simulink library "inp"  (R2021b)
settings: Solver=VariableStepAuto  StartTime=0.0  StopTime=10.0  RelTol=1e-3
undefined symbols (not defined in the file): C_TASK_5MS_S, FALSE, KINP_AcoreReadyToSlp_flg_ovrdflg, KINP_AcoreReadyToSlp_flg_ovrdval, KINP_AllowMovThd_OTA_enum_ovrdflg, KINP_AllowMovThd_OTA_enum_ovrdval, KINP_APSAngleTarget_Deg_ovrdflg, KINP_APSAngleTarget_Deg_ovrdval, KINP_APSDecReq_mps2_ovrdflg, KINP_APSDecReq_mps2_ovrdval, KINP_APSDecReqA_flg_ovrdflg, KINP_APSDecReqA_flg_ovrdval, KINP_APSDFLL_cm_ovrdflg, KINP_APSDFLL_cm_ovrdval, KINP_APSDFLR_cm_ovrdflg, KINP_APSDFLR_cm_ovrdval, KINP_APSDRLL_cm_ovrdflg, KINP_APSDRLL_cm_ovrdval, KINP_APSDRLR_cm_ovrdflg, KINP_APSDRLR_cm_ovrdval, KINP_APSExitCondition_enum_ovrdflg, KINP_APSExitCondition_enum_ovrdval, KINP_APSHWVer_enum_ovrdflg, KINP_APSHWVer_enum_ovrdval, KINP_APSProgressPCT_pct_ovrdflg, KINP_APSProgressPCT_pct_ovrdval, KINP_APSReq_enum_ovrdflg, KINP_APSReq_enum_ovrdval, KINP_APSRQDisplay_enum_ovrdflg, KINP_APSRQDisplay_enum_ovrdval, KINP_APSRqEPASCtrl_flg_ovrdflg, KINP_APSRqEPASCtrl_flg_ovrdval, KINP_APSShiftPosnReq_enum_ovrdval, KINP_APSShiftPosnReq_enum_ovrflg, KINP_APSSpeedCMD_kph_ovrdval, KINP_APSSpeedCMD_kph_ovrflg, KINP_APSStaSystem_enum_ovrdflg, KINP_APSStaSystem_enum_ovrdval, KINP_APSSWVer_enum_ovrdflg, KINP_APSSWVer_enum_ovrdval, KINP_APSVMCReqA_flg_ovrdval, KINP_APSVMCReqA_flg_ovrflg, KINP_APSVRqEPASCtrl_flg_ovrdflg, KINP_APSVRqEPASCtrl_flg_ovrdval, KINP_AuxBattVolmV_mV_ovrdflg, KINP_AuxBattVolmV_mV_ovrdval, KINP_CAASSta_enum_ovrdflg, KINP_CAASSta_enum_ovrdval, KINP_CAASVMCReqA_flg_ovrdval, KINP_CAASVMCReqA_flg_ovrflg, KINP_Chime_enum_ovrdflg, KINP_Chime_enum_ovrdval, KINP_ClearDTCcmd_flg_ovrdflg, KINP_ClearDTCcmd_flg_ovrdval, KINP_EvccAplusPwrUpReq_flg_ovrdflg, KINP_EvccAplusPwrUpReq_flg_ovrdval, KINP_LFID_raw_ovrdval, KINP_LFID_raw_ovrflg, KINP_LRID_raw_ovrdval, KINP_MemOffsetAccX_raw16_ovrdflg ... (+118)
libraries: FVT_lib x595, hcu_lib x1
(part 24 of 27)

== system inp/INP/CAN4/SignalCheck/GW_ZoneFR2 ==
  BHAL_outputs : Inport
  inp_CanValid_bus : Inport  Port=2
  COMPStatorSpd : FVT_lib/inp/can_signal_template  SystemSampleTime=-1  VariantActivationTime=update diagram  Latency=0  AutoFrameSizeCalculation=off
      link override defval: Value=KINP_COMPStatorSpd_rpm_defval
      link override fftdec: Value=KINP_COMPStatorSpd_rpm_fftdec
      link override fftinc: Value=KINP_COMPStatorSpd_rpm_fftinc
      link override fftlim: Value=KINP_COMPStatorSpd_rpm_fftlim
      link override invalid: Value=KINP_COMPStatorSpd_rpm_invalid
      link override ovrdflg: Value=KINP_COMPStatorSpd_rpm_ovrdflg
      link override ovrdval: Value=KINP_COMPStatorSpd_rpm_ovrdval
      link override setvalid: Value=KINP_COMPStatorSpd_rpm_setvalid
      link override srvcflg: Value=KINP_COMPStatorSpd_rpm_srvcflg
      link override srvcval: Value=KINP_COMPStatorSpd_rpm_srvcval
  CompProEN : FVT_lib/inp/can_signal_template  SystemSampleTime=-1  VariantActivationTime=update diagram  Latency=0  AutoFrameSizeCalculation=off
      link override defval: Value=KINP_CompProEN_flg_defval
      link override fftdec: Value=KINP_CompProEN_flg_fftdec
      link override fftinc: Value=KINP_CompProEN_flg_fftinc
      link override fftlim: Value=KINP_CompProEN_flg_fftlim
      link override invalid: Value=KINP_CompProEN_flg_invalid
      link override ovrdflg: Value=KINP_CompProEN_flg_ovrdflg
      link override ovrdval: Value=KINP_CompProEN_flg_ovrdval
      link override setvalid: Value=KINP_CompProEN_flg_setvalid
      link override srvcflg: Value=KINP_CompProEN_flg_srvcflg
      link override srvcval: Value=KINP_CompProEN_flg_srvcval
  Terminator_1 : Terminator
  Terminator_2 : Terminator
  True_VHAL_COMPStatorSpd_rpm : Constant  Value=TRUE  OutDataTypeStr=boolean
  True_VHAL_CompProEN_flg : Constant  Value=TRUE  OutDataTypeStr=boolean
  slr1_1 : BusSelector  OutputSignals=VINP_CANMsgValidGWZoneFR2_flg
  slr1_2 : BusSelector  OutputSignals=VINP_CANMsgValidGWZoneFR2_flg
  slr_VHAL_COMPStatorSpd_rpm : BusSelector  OutputSignals=VHAL_COMPStatorSpd_rpm
  slr_VHAL_CompProEN_flg : BusSelector  OutputSignals=VHAL_CompProEN_flg
  VINP_COMPStatorSpd_rpm : Outport
  VINP_CompProEN_flg : Outport  Port=2
  wires:
  BHAL_outputs/1 -> [BHAL_outputs]
  inp_CanValid_bus/1 -> [inp_CanValid_bus]
  [BHAL_outputs] -> slr_VHAL_COMPStatorSpd_rpm/1
  slr_VHAL_COMPStatorSpd_rpm/1 -> COMPStatorSpd/1  "<VHAL_COMPStatorSpd_rpm>"
  True_VHAL_COMPStatorSpd_rpm/1 -> COMPStatorSpd/2
  [inp_CanValid_bus] -> slr1_1/1
  slr1_1/1 -> COMPStatorSpd/3  "<VINP_CANMsgValidGWZoneFR2_flg>"
  COMPStatorSpd/1 -> VINP_COMPStatorSpd_rpm/1  "VINP_COMPStatorSpd_rpm"
  COMPStatorSpd/2 -> Terminator_1/1
  [BHAL_outputs] -> slr_VHAL_CompProEN_flg/1
  slr_VHAL_CompProEN_flg/1 -> CompProEN/1  "<VHAL_CompProEN_flg>"
  True_VHAL_CompProEN_flg/1 -> CompProEN/2
  [inp_CanValid_bus] -> slr1_2/1
  slr1_2/1 -> CompProEN/3  "<VINP_CANMsgValidGWZoneFR2_flg>"
  CompProEN/1 -> VINP_CompProEN_flg/1  "VINP_CompProEN_flg"
  CompProEN/2 -> Terminator_2/1

== system inp/INP/CAN4/SignalCheck/Zone_Dr_SCP ==
  BHAL_outputs : Inport
  inp_CanValid_bus : Inport  Port=2
  DrSCPSysErrLmp : FVT_lib/inp/can_signal_template  SystemSampleTime=-1  VariantActivationTime=update diagram  Latency=0  AutoFrameSizeCalculation=off
      link override defval: Value=KINP_DrSCPSysErrLmp_flg_defval
      link override fftdec: Value=KINP_DrSCPSysErrLmp_flg_fftdec
      link override fftinc: Value=KINP_DrSCPSysErrLmp_flg_fftinc
      link override fftlim: Value=KINP_DrSCPSysErrLmp_flg_fftlim
      link override invalid: Value=KINP_DrSCPSysErrLmp_flg_invalid
      link override ovrdflg: Value=KINP_DrSCPSysErrLmp_flg_ovrdflg
      link override ovrdval: Value=KINP_DrSCPSysErrLmp_flg_ovrdval
      link override setvalid: Value=KINP_DrSCPSysErrLmp_flg_setvalid
      link override srvcflg: Value=KINP_DrSCPSysErrLmp_flg_srvcflg
      link override srvcval: Value=KINP_DrSCPSysErrLmp_flg_srvcval
  RegenMode : FVT_lib/inp/can_signal_template  SystemSampleTime=-1  VariantActivationTime=update diagram  Latency=0  AutoFrameSizeCalculation=off
      link override defval: Value=KINP_RegenMode_enum_defval
      link override fftdec: Value=KINP_RegenMode_enum_fftdec
      link override fftinc: Value=KINP_RegenMode_enum_fftinc
      link override fftlim: Value=KINP_RegenMode_enum_fftlim
      link override invalid: Value=KINP_RegenMode_enum_invalid
      link override ovrdflg: Value=KINP_RegenMode_enum_ovrdflg
      link override ovrdval: Value=KINP_RegenMode_enum_ovrdval
      link override setvalid: Value=KINP_RegenMode_enum_setvalid
      link override srvcflg: Value=KINP_RegenMode_enum_srvcflg
      link override srvcval: Value=KINP_RegenMode_enum_srvcval
  SetSpd : FVT_lib/inp/can_signal_template  SystemSampleTime=-1  VariantActivationTime=update diagram  Latency=0  AutoFrameSizeCalculation=off
      link override defval: Value=KINP_SetSpd_kph_defval
      link override fftdec: Value=KINP_SetSpd_kph_fftdec
      link override fftinc: Value=KINP_SetSpd_kph_fftinc
      link override fftlim: Value=KINP_SetSpd_kph_fftlim
      link override invalid: Value=KINP_SetSpd_kph_invalid
      link override ovrdflg: Value=KINP_SetSpd_kph_ovrdflg
      link override ovrdval: Value=KINP_SetSpd_kph_ovrdval
      link override setvalid: Value=KINP_SetSpd_kph_setvalid
      link override srvcflg: Value=KINP_SetSpd_kph_srvcflg
      link override srvcval: Value=KINP_SetSpd_kph_srvcval
  Terminator_{1..4} (4 alike) : Terminator
  True_VHAL_DrSCPSysErrLmp_flg : Constant  Value=TRUE  OutDataTypeStr=boolean
  True_VHAL_RegenMode_enum : Constant  Value=TRUE  OutDataTypeStr=boolean
  True_VHAL_SetSpd_kph : Constant  Value=TRUE  OutDataTypeStr=boolean
  True_VHAL_ZoneSpdCtrlMode_enum : Constant  Value=TRUE  OutDataTypeStr=boolean
  ZoneSpdCtrlMode : FVT_lib/inp/can_signal_template  SystemSampleTime=-1  VariantActivationTime=update diagram  Latency=0  AutoFrameSizeCalculation=off
      link override defval: Value=KINP_ZoneSpdCtrlMode_enum_defval
      link override fftdec: Value=KINP_ZoneSpdCtrlMode_enum_fftdec
      link override fftinc: Value=KINP_ZoneSpdCtrlMode_enum_fftinc
      link override fftlim: Value=KINP_ZoneSpdCtrlMode_enum_fftlim
      link override invalid: Value=KINP_ZoneSpdCtrlMode_enum_invalid
      link override ovrdflg: Value=KINP_ZoneSpdCtrlMode_enum_ovrdflg
      link override ovrdval: Value=KINP_ZoneSpdCtrlMode_enum_ovrdval
      link override setvalid: Value=KINP_ZoneSpdCtrlMode_enum_setvalid
      link override srvcflg: Value=KINP_ZoneSpdCtrlMode_enum_srvcflg
      link override srvcval: Value=KINP_ZoneSpdCtrlMode_enum_srvcval
  slr1_{1..4} (4 alike) : BusSelector  OutputSignals=VINP_CANMsgValidZoneDrSCP_flg
  slr_VHAL_DrSCPSysErrLmp_flg : BusSelector  OutputSignals=VHAL_DrSCPSysErrLmp_flg
  slr_VHAL_RegenMode_enum : BusSelector  OutputSignals=VHAL_RegenMode_enum
  slr_VHAL_SetSpd_kph : BusSelector  OutputSignals=VHAL_SetSpd_kph
  slr_VHAL_ZoneSpdCtrlMode_enum : BusSelector  OutputSignals=VHAL_ZoneSpdCtrlMode_enum
  VINP_DrSCPSysErrLmp_flg : Outport
  VINP_RegenMode_enum : Outport  Port=2
  VINP_SetSpd_kph : Outport  Port=3
  VINP_ZoneSpdCtrlMode_enum : Outport  Port=4
  wires:
  BHAL_outputs/1 -> [BHAL_outputs]
  inp_CanValid_bus/1 -> [inp_CanValid_bus]
  [BHAL_outputs] -> slr_VHAL_DrSCPSysErrLmp_flg/1
  slr_VHAL_DrSCPSysErrLmp_flg/1 -> DrSCPSysErrLmp/1  "<VHAL_DrSCPSysErrLmp_flg>"
  True_VHAL_DrSCPSysErrLmp_flg/1 -> DrSCPSysErrLmp/2
  [inp_CanValid_bus] -> slr1_1/1
  slr1_1/1 -> DrSCPSysErrLmp/3  "<VINP_CANMsgValidZoneDrSCP_flg>"
  DrSCPSysErrLmp/1 -> VINP_DrSCPSysErrLmp_flg/1  "VINP_DrSCPSysErrLmp_flg"
  DrSCPSysErrLmp/2 -> Terminator_1/1
  [BHAL_outputs] -> slr_VHAL_RegenMode_enum/1
  slr_VHAL_RegenMode_enum/1 -> RegenMode/1  "<VHAL_RegenMode_enum>"
  True_VHAL_RegenMode_enum/1 -> RegenMode/2
  [inp_CanValid_bus] -> slr1_2/1
  slr1_2/1 -> RegenMode/3  "<VINP_CANMsgValidZoneDrSCP_flg>"
  RegenMode/1 -> VINP_RegenMode_enum/1  "VINP_RegenMode_enum"
  RegenMode/2 -> Terminator_2/1
  [BHAL_outputs] -> slr_VHAL_SetSpd_kph/1
  slr_VHAL_SetSpd_kph/1 -> SetSpd/1  "<VHAL_SetSpd_kph>"
  True_VHAL_SetSpd_kph/1 -> SetSpd/2
  [inp_CanValid_bus] -> slr1_3/1
  slr1_3/1 -> SetSpd/3  "<VINP_CANMsgValidZoneDrSCP_flg>"
  SetSpd/1 -> VINP_SetSpd_kph/1  "VINP_SetSpd_kph"
  SetSpd/2 -> Terminator_3/1
  [BHAL_outputs] -> slr_VHAL_ZoneSpdCtrlMode_enum/1
  slr_VHAL_ZoneSpdCtrlMode_enum/1 -> ZoneSpdCtrlMode/1  "<VHAL_ZoneSpdCtrlMode_enum>"
  True_VHAL_ZoneSpdCtrlMode_enum/1 -> ZoneSpdCtrlMode/2
  [inp_CanValid_bus] -> slr1_4/1
  slr1_4/1 -> ZoneSpdCtrlMode/3  "<VINP_CANMsgValidZoneDrSCP_flg>"
  ZoneSpdCtrlMode/1 -> VINP_ZoneSpdCtrlMode_enum/1  "VINP_ZoneSpdCtrlMode_enum"
  ZoneSpdCtrlMode/2 -> Terminator_4/1

== system inp/INP/CAN4/SignalCheck/Zone_Dr_THCM ==
  BHAL_outputs : Inport
  inp_CanValid_bus : Inport  Port=2
  BlowerErr : FVT_lib/inp/can_signal_template  SystemSampleTime=-1  VariantActivationTime=update diagram  Latency=0  AutoFrameSizeCalculation=off
      link override defval: Value=KINP_BlowerErr_enum_defval
      link override fftdec: Value=KINP_BlowerErr_enum_fftdec
      link override fftinc: Value=KINP_BlowerErr_enum_fftinc
      link override fftlim: Value=KINP_BlowerErr_enum_fftlim
      link override invalid: Value=KINP_BlowerErr_enum_invalid
      link override ovrdflg: Value=KINP_BlowerErr_enum_ovrdflg
      link override ovrdval: Value=KINP_BlowerErr_enum_ovrdval
      link override setvalid: Value=KINP_BlowerErr_enum_setvalid
      link override srvcflg: Value=KINP_BlowerErr_enum_srvcflg
      link override srvcval: Value=KINP_BlowerErr_enum_srvcval
  SolarL : FVT_lib/inp/can_signal_template  SystemSampleTime=-1  VariantActivationTime=update diagram  Latency=0  AutoFrameSizeCalculation=off
      link override defval: Value=KINP_SolarL_W_defval
      link override fftdec: Value=KINP_SolarL_W_fftdec
      link override fftinc: Value=KINP_SolarL_W_fftinc
      link override fftlim: Value=KINP_SolarL_W_fftlim
      link override invalid: Value=KINP_SolarL_W_invalid
      link override ovrdflg: Value=KINP_SolarL_W_ovrdflg
      link override ovrdval: Value=KINP_SolarL_W_ovrdval
      link override setvalid: Value=KINP_SolarL_W_setvalid
      link override srvcflg: Value=KINP_SolarL_W_srvcflg
      link override srvcval: Value=KINP_SolarL_W_srvcval
  SolarLErr : FVT_lib/inp/can_signal_template  SystemSampleTime=-1  VariantActivationTime=update diagram  Latency=0  AutoFrameSizeCalculation=off
      link override defval: Value=KINP_SolarLErr_enum_defval
      link override fftdec: Value=KINP_SolarLErr_enum_fftdec
      link override fftinc: Value=KINP_SolarLErr_enum_fftinc
      link override fftlim: Value=KINP_SolarLErr_enum_fftlim
      link override invalid: Value=KINP_SolarLErr_enum_invalid
      link override ovrdflg: Value=KINP_SolarLErr_enum_ovrdflg
      link override ovrdval: Value=KINP_SolarLErr_enum_ovrdval
      link override setvalid: Value=KINP_SolarLErr_enum_setvalid
      link override srvcflg: Value=KINP_SolarLErr_enum_srvcflg
      link override srvcval: Value=KINP_SolarLErr_enum_srvcval
  SolarR : FVT_lib/inp/can_signal_template  SystemSampleTime=-1  VariantActivationTime=update diagram  Latency=0  AutoFrameSizeCalculation=off
      link override defval: Value=KINP_SolarR_W_defval
      link override fftdec: Value=KINP_SolarR_W_fftdec
      link override fftinc: Value=KINP_SolarR_W_fftinc
      link override fftlim: Value=KINP_SolarR_W_fftlim
      link override invalid: Value=KINP_SolarR_W_invalid
      link override ovrdflg: Value=KINP_SolarR_W_ovrdflg
      link override ovrdval: Value=KINP_SolarR_W_ovrdval
      link override setvalid: Value=KINP_SolarR_W_setvalid
      link override srvcflg: Value=KINP_SolarR_W_srvcflg
      link override srvcval: Value=KINP_SolarR_W_srvcval
  SolarRErr : FVT_lib/inp/can_signal_template  SystemSampleTime=-1  VariantActivationTime=update diagram  Latency=0  AutoFrameSizeCalculation=off
      link override defval: Value=KINP_SolarRErr_enum_defval
      link override fftdec: Value=KINP_SolarRErr_enum_fftdec
      link override fftinc: Value=KINP_SolarRErr_enum_fftinc
      link override fftlim: Value=KINP_SolarRErr_enum_fftlim
      link override invalid: Value=KINP_SolarRErr_enum_invalid
      link override ovrdflg: Value=KINP_SolarRErr_enum_ovrdflg
      link override ovrdval: Value=KINP_SolarRErr_enum_ovrdval
      link override setvalid: Value=KINP_SolarRErr_enum_setvalid
      link override srvcflg: Value=KINP_SolarRErr_enum_srvcflg
      link override srvcval: Value=KINP_SolarRErr_enum_srvcval
  TFaceL : FVT_lib/inp/can_signal_template  SystemSampleTime=-1  VariantActivationTime=update diagram  Latency=0  AutoFrameSizeCalculation=off
      link override defval: Value=KINP_TFaceL_C_defval
      link override fftdec: Value=KINP_TFaceL_C_fftdec
      link override fftinc: Value=KINP_TFaceL_C_fftinc
      link override fftlim: Value=KINP_TFaceL_C_fftlim
      link override invalid: Value=KINP_TFaceL_C_invalid
      link override ovrdflg: Value=KINP_TFaceL_C_ovrdflg
      link override ovrdval: Value=KINP_TFaceL_C_ovrdval
      link override setvalid: Value=KINP_TFaceL_C_setvalid
      link override srvcflg: Value=KINP_TFaceL_C_srvcflg
      link override srvcval: Value=KINP_TFaceL_C_srvcval
  TFaceLErr : FVT_lib/inp/can_signal_template  SystemSampleTime=-1  VariantActivationTime=update diagram  Latency=0  AutoFrameSizeCalculation=off
      link override defval: Value=KINP_TFaceLErr_enum_defval
      link override fftdec: Value=KINP_TFaceLErr_enum_fftdec
      link override fftinc: Value=KINP_TFaceLErr_enum_fftinc
      link override fftlim: Value=KINP_TFaceLErr_enum_fftlim
      link override invalid: Value=KINP_TFaceLErr_enum_invalid
      link override ovrdflg: Value=KINP_TFaceLErr_enum_ovrdflg
      link override ovrdval: Value=KINP_TFaceLErr_enum_ovrdval
      link override setvalid: Value=KINP_TFaceLErr_enum_setvalid
      link override srvcflg: Value=KINP_TFaceLErr_enum_srvcflg
      link override srvcval: Value=KINP_TFaceLErr_enum_srvcval
  TFaceR : FVT_lib/inp/can_signal_template  SystemSampleTime=-1  VariantActivationTime=update diagram  Latency=0  AutoFrameSizeCalculation=off
      link override defval: Value=KINP_TFaceR_C_defval
      link override fftdec: Value=KINP_TFaceR_C_fftdec
      link override fftinc: Value=KINP_TFaceR_C_fftinc
      link override fftlim: Value=KINP_TFaceR_C_fftlim
      link override invalid: Value=KINP_TFaceR_C_invalid
      link override ovrdflg: Value=KINP_TFaceR_C_ovrdflg
      link override ovrdval: Value=KINP_TFaceR_C_ovrdval
      link override setvalid: Value=KINP_TFaceR_C_setvalid
      link override srvcflg: Value=KINP_TFaceR_C_srvcflg
      link override srvcval: Value=KINP_TFaceR_C_srvcval
  TFaceRErr : FVT_lib/inp/can_signal_template  SystemSampleTime=-1  VariantActivationTime=update diagram  Latency=0  AutoFrameSizeCalculation=off
      link override defval: Value=KINP_TFaceRErr_enum_defval
      link override fftdec: Value=KINP_TFaceRErr_enum_fftdec
      link override fftinc: Value=KINP_TFaceRErr_enum_fftinc
      link override fftlim: Value=KINP_TFaceRErr_enum_fftlim
      link override invalid: Value=KINP_TFaceRErr_enum_invalid
      link override ovrdflg: Value=KINP_TFaceRErr_enum_ovrdflg
      link override ovrdval: Value=KINP_TFaceRErr_enum_ovrdval
      link override setvalid: Value=KINP_TFaceRErr_enum_setvalid
      link override srvcflg: Value=KINP_TFaceRErr_enum_srvcflg
      link override srvcval: Value=KINP_TFaceRErr_enum_srvcval
  TFaceRr : FVT_lib/inp/can_signal_template  SystemSampleTime=-1  VariantActivationTime=update diagram  Latency=0  AutoFrameSizeCalculation=off
      link override defval: Value=KINP_TFaceRr_C_defval
      link override fftdec: Value=KINP_TFaceRr_C_fftdec
      link override fftinc: Value=KINP_TFaceRr_C_fftinc
      link override fftlim: Value=KINP_TFaceRr_C_fftlim
      link override invalid: Value=KINP_TFaceRr_C_invalid
      link override ovrdflg: Value=KINP_TFaceRr_C_ovrdflg
      link override ovrdval: Value=KINP_TFaceRr_C_ovrdval
      link override setvalid: Value=KINP_TFaceRr_C_setvalid
      link override srvcflg: Value=KINP_TFaceRr_C_srvcflg
      link override srvcval: Value=KINP_TFaceRr_C_srvcval
  TFaceRrErr : FVT_lib/inp/can_signal_template  SystemSampleTime=-1  VariantActivationTime=update diagram  Latency=0  AutoFrameSizeCalculation=off
      link override defval: Value=KINP_TFaceRrErr_enum_defval
      link override fftdec: Value=KINP_TFaceRrErr_enum_fftdec
      link override fftinc: Value=KINP_TFaceRrErr_enum_fftinc
      link override fftlim: Value=KINP_TFaceRrErr_enum_fftlim
      link override invalid: Value=KINP_TFaceRrErr_enum_invalid
      link override ovrdflg: Value=KINP_TFaceRrErr_enum_ovrdflg
      link override ovrdval: Value=KINP_TFaceRrErr_enum_ovrdval
      link override setvalid: Value=KINP_TFaceRrErr_enum_setvalid
      link override srvcflg: Value=KINP_TFaceRrErr_enum_srvcflg
      link override srvcval: Value=KINP_TFaceRrErr_enum_srvcval
  TFootL : FVT_lib/inp/can_signal_template  SystemSampleTime=-1  VariantActivationTime=update diagram  Latency=0  AutoFrameSizeCalculation=off
      link override defval: Value=KINP_TFootL_C_defval
      link override fftdec: Value=KINP_TFootL_C_fftdec
      link override fftinc: Value=KINP_TFootL_C_fftinc
      link override fftlim: Value=KINP_TFootL_C_fftlim
      link override invalid: Value=KINP_TFootL_C_invalid
      link override ovrdflg: Value=KINP_TFootL_C_ovrdflg
      link override ovrdval: Value=KINP_TFootL_C_ovrdval
      link override setvalid: Value=KINP_TFootL_C_setvalid
      link override srvcflg: Value=KINP_TFootL_C_srvcflg
      link override srvcval: Value=KINP_TFootL_C_srvcval
  TFootLErr : FVT_lib/inp/can_signal_template  SystemSampleTime=-1  VariantActivationTime=update diagram  Latency=0  AutoFrameSizeCalculation=off
      link override defval: Value=KINP_TFootLErr_enum_defval
      link override fftdec: Value=KINP_TFootLErr_enum_fftdec
      link override fftinc: Value=KINP_TFootLErr_enum_fftinc
      link override fftlim: Value=KINP_TFootLErr_enum_fftlim
      link override invalid: Value=KINP_TFootLErr_enum_invalid
      link override ovrdflg: Value=KINP_TFootLErr_enum_ovrdflg
      link override ovrdval: Value=KINP_TFootLErr_enum_ovrdval
      link override setvalid: Value=KINP_TFootLErr_enum_setvalid
      link override srvcflg: Value=KINP_TFootLErr_enum_srvcflg
      link override srvcval: Value=KINP_TFootLErr_enum_srvcval
  TFootR : FVT_lib/inp/can_signal_template  SystemSampleTime=-1  VariantActivationTime=update diagram  Latency=0  AutoFrameSizeCalculation=off
      link override defval: Value=KINP_TFootR_C_defval
      link override fftdec: Value=KINP_TFootR_C_fftdec
      link override fftinc: Value=KINP_TFootR_C_fftinc
      link override fftlim: Value=KINP_TFootR_C_fftlim
      link override invalid: Value=KINP_TFootR_C_invalid
      link override ovrdflg: Value=KINP_TFootR_C_ovrdflg
      link override ovrdval: Value=KINP_TFootR_C_ovrdval
      link override setvalid: Value=KINP_TFootR_C_setvalid
      link override srvcflg: Value=KINP_TFootR_C_srvcflg
      link override srvcval: Value=KINP_TFootR_C_srvcval
  TFootRErr : FVT_lib/inp/can_signal_template  SystemSampleTime=-1  VariantActivationTime=update diagram  Latency=0  AutoFrameSizeCalculation=off
      link override defval: Value=KINP_TFootRErr_enum_defval
      link override fftdec: Value=KINP_TFootRErr_enum_fftdec
      link override fftinc: Value=KINP_TFootRErr_enum_fftinc
      link override fftlim: Value=KINP_TFootRErr_enum_fftlim
      link override invalid: Value=KINP_TFootRErr_enum_invalid
      link override ovrdflg: Value=KINP_TFootRErr_enum_ovrdflg
      link override ovrdval: Value=KINP_TFootRErr_enum_ovrdval
      link override setvalid: Value=KINP_TFootRErr_enum_setvalid
      link override srvcflg: Value=KINP_TFootRErr_enum_srvcflg
      link override srvcval: Value=KINP_TFootRErr_enum_srvcval
  TFootRr : FVT_lib/inp/can_signal_template  SystemSampleTime=-1  VariantActivationTime=update diagram  Latency=0  AutoFrameSizeCalculation=off
      link override defval: Value=KINP_TFootRr_C_defval
      link override fftdec: Value=KINP_TFootRr_C_fftdec
      link override fftinc: Value=KINP_TFootRr_C_fftinc
      link override fftlim: Value=KINP_TFootRr_C_fftlim
      link override invalid: Value=KINP_TFootRr_C_invalid
      link override ovrdflg: Value=KINP_TFootRr_C_ovrdflg
      link override ovrdval: Value=KINP_TFootRr_C_ovrdval
      link override setvalid: Value=KINP_TFootRr_C_setvalid
      link override srvcflg: Value=KINP_TFootRr_C_srvcflg
      link override srvcval: Value=KINP_TFootRr_C_srvcval
  TFootRrErr : FVT_lib/inp/can_signal_template  SystemSampleTime=-1  VariantActivationTime=update diagram  Latency=0  AutoFrameSizeCalculation=off
      link override defval: Value=KINP_TFootRrErr_enum_defval
      link override fftdec: Value=KINP_TFootRrErr_enum_fftdec
      link override fftinc: Value=KINP_TFootRrErr_enum_fftinc
      link override fftlim: Value=KINP_TFootRrErr_enum_fftlim
      link override invalid: Value=KINP_TFootRrErr_enum_invalid
      link override ovrdflg: Value=KINP_TFootRrErr_enum_ovrdflg
      link override ovrdval: Value=KINP_TFootRrErr_enum_ovrdval
      link override setvalid: Value=KINP_TFootRrErr_enum_setvalid
      link override srvcflg: Value=KINP_TFootRrErr_enum_srvcflg
      link override srvcval: Value=KINP_TFootRrErr_enum_srvcval
  Terminator_{1..21} (21 alike) : Terminator
  Tevap : FVT_lib/inp/can_signal_template  SystemSampleTime=-1  VariantActivationTime=update diagram  Latency=0  AutoFrameSizeCalculation=off
      link override defval: Value=KINP_Tevap_C_defval
      link override fftdec: Value=KINP_Tevap_C_fftdec
      link override fftinc: Value=KINP_Tevap_C_fftinc
      link override fftlim: Value=KINP_Tevap_C_fftlim
      link override invalid: Value=KINP_Tevap_C_invalid
      link override ovrdflg: Value=KINP_Tevap_C_ovrdflg
      link override ovrdval: Value=KINP_Tevap_C_ovrdval
      link override setvalid: Value=KINP_Tevap_C_setvalid
      link override srvcflg: Value=KINP_Tevap_C_srvcflg
      link override srvcval: Value=KINP_Tevap_C_srvcval
  TevapErr : FVT_lib/inp/can_signal_template  SystemSampleTime=-1  VariantActivationTime=update diagram  Latency=0  AutoFrameSizeCalculation=off
      link override defval: Value=KINP_TevapErr_enum_defval
      link override fftdec: Value=KINP_TevapErr_enum_fftdec
      link override fftinc: Value=KINP_TevapErr_enum_fftinc
      link override fftlim: Value=KINP_TevapErr_enum_fftlim
      link override invalid: Value=KINP_TevapErr_enum_invalid
      link override ovrdflg: Value=KINP_TevapErr_enum_ovrdflg
      link override ovrdval: Value=KINP_TevapErr_enum_ovrdval
      link override setvalid: Value=KINP_TevapErr_enum_setvalid
      link override srvcflg: Value=KINP_TevapErr_enum_srvcflg
      link override srvcval: Value=KINP_TevapErr_enum_srvcval
  Tincar : FVT_lib/inp/can_signal_template  SystemSampleTime=-1  VariantActivationTime=update diagram  Latency=0  AutoFrameSizeCalculation=off
      link override defval: Value=KINP_Tincar_C_defval
      link override fftdec: Value=KINP_Tincar_C_fftdec
      link override fftinc: Value=KINP_Tincar_C_fftinc
      link override fftlim: Value=KINP_Tincar_C_fftlim
      link override invalid: Value=KINP_Tincar_C_invalid
      link override ovrdflg: Value=KINP_Tincar_C_ovrdflg
      link override ovrdval: Value=KINP_Tincar_C_ovrdval
      link override setvalid: Value=KINP_Tincar_C_setvalid
      link override srvcflg: Value=KINP_Tincar_C_srvcflg
      link override srvcval: Value=KINP_Tincar_C_srvcval
  TincarErr : FVT_lib/inp/can_signal_template  SystemSampleTime=-1  VariantActivationTime=update diagram  Latency=0  AutoFrameSizeCalculation=off
      link override defval: Value=KINP_TincarErr_enum_defval
      link override fftdec: Value=KINP_TincarErr_enum_fftdec
      link override fftinc: Value=KINP_TincarErr_enum_fftinc
      link override fftlim: Value=KINP_TincarErr_enum_fftlim
      link override invalid: Value=KINP_TincarErr_enum_invalid
      link override ovrdflg: Value=KINP_TincarErr_enum_ovrdflg
      link override ovrdval: Value=KINP_TincarErr_enum_ovrdval
      link override setvalid: Value=KINP_TincarErr_enum_setvalid
      link override srvcflg: Value=KINP_TincarErr_enum_srvcflg
      link override srvcval: Value=KINP_TincarErr_enum_srvcval
  True_VHAL_BlowerErr_enum : Constant  Value=TRUE  OutDataTypeStr=boolean
  True_VHAL_SolarLErr_enum : Constant  Value=TRUE  OutDataTypeStr=boolean
  True_VHAL_SolarL_W : Constant  Value=TRUE  OutDataTypeStr=boolean
  True_VHAL_SolarRErr_enum : Constant  Value=TRUE  OutDataTypeStr=boolean
  True_VHAL_SolarR_W : Constant  Value=TRUE  OutDataTypeStr=boolean
  True_VHAL_TFaceLErr_enum : Constant  Value=TRUE  OutDataTypeStr=boolean
  True_VHAL_TFaceL_C : Constant  Value=TRUE  OutDataTypeStr=boolean
  True_VHAL_TFaceRErr_enum : Constant  Value=TRUE  OutDataTypeStr=boolean
  True_VHAL_TFaceR_C : Constant  Value=TRUE  OutDataTypeStr=boolean
  True_VHAL_TFaceRrErr_enum : Constant  Value=TRUE  OutDataTypeStr=boolean
  True_VHAL_TFaceRr_C : Constant  Value=TRUE  OutDataTypeStr=boolean
  True_VHAL_TFootLErr_enum : Constant  Value=TRUE  OutDataTypeStr=boolean
  True_VHAL_TFootL_C : Constant  Value=TRUE  OutDataTypeStr=boolean
  True_VHAL_TFootRErr_enum : Constant  Value=TRUE  OutDataTypeStr=boolean
  True_VHAL_TFootR_C : Constant  Value=TRUE  OutDataTypeStr=boolean
  True_VHAL_TFootRrErr_enum : Constant  Value=TRUE  OutDataTypeStr=boolean
  True_VHAL_TFootRr_C : Constant  Value=TRUE  OutDataTypeStr=boolean
  True_VHAL_TevapErr_enum : Constant  Value=TRUE  OutDataTypeStr=boolean
  True_VHAL_Tevap_C : Constant  Value=TRUE  OutDataTypeStr=boolean
  True_VHAL_TincarErr_enum : Constant  Value=TRUE  OutDataTypeStr=boolean
  True_VHAL_Tincar_C : Constant  Value=TRUE  OutDataTypeStr=boolean
  slr1_{1..21} (21 alike) : BusSelector  OutputSignals=VINP_CANMsgValidZoneDrTHCM_flg
  slr_VHAL_BlowerErr_enum : BusSelector  OutputSignals=VHAL_BlowerErr_enum
  slr_VHAL_SolarLErr_enum : BusSelector  OutputSignals=VHAL_SolarLErr_enum
  slr_VHAL_SolarL_W : BusSelector  OutputSignals=VHAL_SolarL_W
  slr_VHAL_SolarRErr_enum : BusSelector  OutputSignals=VHAL_SolarRErr_enum
  slr_VHAL_SolarR_W : BusSelector  OutputSignals=VHAL_SolarR_W
  slr_VHAL_TFaceLErr_enum : BusSelector  OutputSignals=VHAL_TFaceLErr_enum
  slr_VHAL_TFaceL_C : BusSelector  OutputSignals=VHAL_TFaceL_C
  slr_VHAL_TFaceRErr_enum : BusSelector  OutputSignals=VHAL_TFaceRErr_enum
  slr_VHAL_TFaceR_C : BusSelector  OutputSignals=VHAL_TFaceR_C
  slr_VHAL_TFaceRrErr_enum : BusSelector  OutputSignals=VHAL_TFaceRrErr_enum
  slr_VHAL_TFaceRr_C : BusSelector  OutputSignals=VHAL_TFaceRr_C
  slr_VHAL_TFootLErr_enum : BusSelector  OutputSignals=VHAL_TFootLErr_enum
  slr_VHAL_TFootL_C : BusSelector  OutputSignals=VHAL_TFootL_C
  slr_VHAL_TFootRErr_enum : BusSelector  OutputSignals=VHAL_TFootRErr_enum
  slr_VHAL_TFootR_C : BusSelector  OutputSignals=VHAL_TFootR_C
  slr_VHAL_TFootRrErr_enum : BusSelector  OutputSignals=VHAL_TFootRrErr_enum
  slr_VHAL_TFootRr_C : BusSelector  OutputSignals=VHAL_TFootRr_C
  slr_VHAL_TevapErr_enum : BusSelector  OutputSignals=VHAL_TevapErr_enum
  slr_VHAL_Tevap_C : BusSelector  OutputSignals=VHAL_Tevap_C
  slr_VHAL_TincarErr_enum : BusSelector  OutputSignals=VHAL_TincarErr_enum
  slr_VHAL_Tincar_C : BusSelector  OutputSignals=VHAL_Tincar_C
  VINP_BlowerErr_enum : Outport
  VINP_SolarL_W : Outport  Port=2
  VINP_SolarLErr_enum : Outport  Port=3
  VINP_SolarR_W : Outport  Port=4
  VINP_SolarRErr_enum : Outport  Port=5
  VINP_TFaceL_C : Outport  Port=6
  VINP_TFaceLErr_enum : Outport  Port=7
  VINP_TFaceR_C : Outport  Port=8
  VINP_TFaceRErr_enum : Outport  Port=9
  VINP_TFaceRr_C : Outport  Port=10
  VINP_TFaceRrErr_enum : Outport  Port=11
  VINP_TFootL_C : Outport  Port=12
  VINP_TFootLErr_enum : Outport  Port=13
  VINP_TFootR_C : Outport  Port=14
  VINP_TFootRErr_enum : Outport  Port=15
  VINP_TFootRr_C : Outport  Port=16
  VINP_TFootRrErr_enum : Outport  Port=17
  VINP_Tevap_C : Outport  Port=18
  VINP_TevapErr_enum : Outport  Port=19
  VINP_Tincar_C : Outport  Port=20
  VINP_TincarErr_enum : Outport  Port=21
  wires:
  BHAL_outputs/1 -> [BHAL_outputs]
  inp_CanValid_bus/1 -> [inp_CanValid_bus]
  [BHAL_outputs] -> slr_VHAL_BlowerErr_enum/1
  slr_VHAL_BlowerErr_enum/1 -> BlowerErr/1  "<VHAL_BlowerErr_enum>"
  True_VHAL_BlowerErr_enum/1 -> BlowerErr/2
  [inp_CanValid_bus] -> slr1_1/1
  slr1_1/1 -> BlowerErr/3  "<VINP_CANMsgValidZoneDrTHCM_flg>"
  BlowerErr/1 -> VINP_BlowerErr_enum/1  "VINP_BlowerErr_enum"
  BlowerErr/2 -> Terminator_1/1
  [BHAL_outputs] -> slr_VHAL_SolarL_W/1
  slr_VHAL_SolarL_W/1 -> SolarL/1  "<VHAL_SolarL_W>"
  True_VHAL_SolarL_W/1 -> SolarL/2
  [inp_CanValid_bus] -> slr1_2/1
  slr1_2/1 -> SolarL/3  "<VINP_CANMsgValidZoneDrTHCM_flg>"
  SolarL/1 -> VINP_SolarL_W/1  "VINP_SolarL_W"
  SolarL/2 -> Terminator_2/1
  [BHAL_outputs] -> slr_VHAL_SolarLErr_enum/1
  slr_VHAL_SolarLErr_enum/1 -> SolarLErr/1  "<VHAL_SolarLErr_enum>"
  True_VHAL_SolarLErr_enum/1 -> SolarLErr/2
  [inp_CanValid_bus] -> slr1_3/1
  slr1_3/1 -> SolarLErr/3  "<VINP_CANMsgValidZoneDrTHCM_flg>"
  SolarLErr/1 -> VINP_SolarLErr_enum/1  "VINP_SolarLErr_enum"
  SolarLErr/2 -> Terminator_3/1
  [BHAL_outputs] -> slr_VHAL_SolarR_W/1
  slr_VHAL_SolarR_W/1 -> SolarR/1  "<VHAL_SolarR_W>"
  True_VHAL_SolarR_W/1 -> SolarR/2
  [inp_CanValid_bus] -> slr1_4/1
  slr1_4/1 -> SolarR/3  "<VINP_CANMsgValidZoneDrTHCM_flg>"
  SolarR/1 -> VINP_SolarR_W/1  "VINP_SolarR_W"
  SolarR/2 -> Terminator_4/1
  [BHAL_outputs] -> slr_VHAL_SolarRErr_enum/1
  slr_VHAL_SolarRErr_enum/1 -> SolarRErr/1  "<VHAL_SolarRErr_enum>"
  True_VHAL_SolarRErr_enum/1 -> SolarRErr/2
  [inp_CanValid_bus] -> slr1_5/1
  slr1_5/1 -> SolarRErr/3  "<VINP_CANMsgValidZoneDrTHCM_flg>"
  SolarRErr/1 -> VINP_SolarRErr_enum/1  "VINP_SolarRErr_enum"
  SolarRErr/2 -> Terminator_5/1
  [BHAL_outputs] -> slr_VHAL_TFaceL_C/1
  slr_VHAL_TFaceL_C/1 -> TFaceL/1  "<VHAL_TFaceL_C>"
  True_VHAL_TFaceL_C/1 -> TFaceL/2
  [inp_CanValid_bus] -> slr1_6/1
  slr1_6/1 -> TFaceL/3  "<VINP_CANMsgValidZoneDrTHCM_flg>"
  TFaceL/1 -> VINP_TFaceL_C/1  "VINP_TFaceL_C"
  TFaceL/2 -> Terminator_6/1
  [BHAL_outputs] -> slr_VHAL_TFaceLErr_enum/1
  slr_VHAL_TFaceLErr_enum/1 -> TFaceLErr/1  "<VHAL_TFaceLErr_enum>"
  True_VHAL_TFaceLErr_enum/1 -> TFaceLErr/2
  [inp_CanValid_bus] -> slr1_7/1
  slr1_7/1 -> TFaceLErr/3  "<VINP_CANMsgValidZoneDrTHCM_flg>"
  TFaceLErr/1 -> VINP_TFaceLErr_enum/1  "VINP_TFaceLErr_enum"
  TFaceLErr/2 -> Terminator_7/1
  [BHAL_outputs] -> slr_VHAL_TFaceR_C/1
  slr_VHAL_TFaceR_C/1 -> TFaceR/1  "<VHAL_TFaceR_C>"
  True_VHAL_TFaceR_C/1 -> TFaceR/2
  [inp_CanValid_bus] -> slr1_8/1
  slr1_8/1 -> TFaceR/3  "<VINP_CANMsgValidZoneDrTHCM_flg>"
  TFaceR/1 -> VINP_TFaceR_C/1  "VINP_TFaceR_C"
  TFaceR/2 -> Terminator_8/1
  [BHAL_outputs] -> slr_VHAL_TFaceRErr_enum/1
  slr_VHAL_TFaceRErr_enum/1 -> TFaceRErr/1  "<VHAL_TFaceRErr_enum>"
  True_VHAL_TFaceRErr_enum/1 -> TFaceRErr/2
  [inp_CanValid_bus] -> slr1_9/1
  slr1_9/1 -> TFaceRErr/3  "<VINP_CANMsgValidZoneDrTHCM_flg>"
  TFaceRErr/1 -> VINP_TFaceRErr_enum/1  "VINP_TFaceRErr_enum"
  TFaceRErr/2 -> Terminator_9/1
  [BHAL_outputs] -> slr_VHAL_TFaceRr_C/1
  slr_VHAL_TFaceRr_C/1 -> TFaceRr/1  "<VHAL_TFaceRr_C>"
  True_VHAL_TFaceRr_C/1 -> TFaceRr/2
  [inp_CanValid_bus] -> slr1_10/1
  slr1_10/1 -> TFaceRr/3  "<VINP_CANMsgValidZoneDrTHCM_flg>"
  TFaceRr/1 -> VINP_TFaceRr_C/1  "VINP_TFaceRr_C"
  TFaceRr/2 -> Terminator_10/1
  [BHAL_outputs] -> slr_VHAL_TFaceRrErr_enum/1
  slr_VHAL_TFaceRrErr_enum/1 -> TFaceRrErr/1  "<VHAL_TFaceRrErr_enum>"
  True_VHAL_TFaceRrErr_enum/1 -> TFaceRrErr/2
  [inp_CanValid_bus] -> slr1_11/1
  slr1_11/1 -> TFaceRrErr/3  "<VINP_CANMsgValidZoneDrTHCM_flg>"
  TFaceRrErr/1 -> VINP_TFaceRrErr_enum/1  "VINP_TFaceRrErr_enum"
  TFaceRrErr/2 -> Terminator_11/1
  [BHAL_outputs] -> slr_VHAL_TFootL_C/1
  slr_VHAL_TFootL_C/1 -> TFootL/1  "<VHAL_TFootL_C>"
  True_VHAL_TFootL_C/1 -> TFootL/2
  [inp_CanValid_bus] -> slr1_12/1
  slr1_12/1 -> TFootL/3  "<VINP_CANMsgValidZoneDrTHCM_flg>"
  TFootL/1 -> VINP_TFootL_C/1  "VINP_TFootL_C"
  TFootL/2 -> Terminator_12/1
  [BHAL_outputs] -> slr_VHAL_TFootLErr_enum/1
  slr_VHAL_TFootLErr_enum/1 -> TFootLErr/1  "<VHAL_TFootLErr_enum>"
  True_VHAL_TFootLErr_enum/1 -> TFootLErr/2
  [inp_CanValid_bus] -> slr1_13/1
  slr1_13/1 -> TFootLErr/3  "<VINP_CANMsgValidZoneDrTHCM_flg>"
  TFootLErr/1 -> VINP_TFootLErr_enum/1  "VINP_TFootLErr_enum"
  TFootLErr/2 -> Terminator_13/1
  [BHAL_outputs] -> slr_VHAL_TFootR_C/1
  slr_VHAL_TFootR_C/1 -> TFootR/1  "<VHAL_TFootR_C>"
  True_VHAL_TFootR_C/1 -> TFootR/2
  [inp_CanValid_bus] -> slr1_14/1
  slr1_14/1 -> TFootR/3  "<VINP_CANMsgValidZoneDrTHCM_flg>"
  TFootR/1 -> VINP_TFootR_C/1  "VINP_TFootR_C"
  TFootR/2 -> Terminator_14/1
  [BHAL_outputs] -> slr_VHAL_TFootRErr_enum/1
  slr_VHAL_TFootRErr_enum/1 -> TFootRErr/1  "<VHAL_TFootRErr_enum>"
  True_VHAL_TFootRErr_enum/1 -> TFootRErr/2
  [inp_CanValid_bus] -> slr1_15/1
  slr1_15/1 -> TFootRErr/3  "<VINP_CANMsgValidZoneDrTHCM_flg>"
  TFootRErr/1 -> VINP_TFootRErr_enum/1  "VINP_TFootRErr_enum"
  TFootRErr/2 -> Terminator_15/1
  [BHAL_outputs] -> slr_VHAL_TFootRr_C/1
  slr_VHAL_TFootRr_C/1 -> TFootRr/1  "<VHAL_TFootRr_C>"
  True_VHAL_TFootRr_C/1 -> TFootRr/2
  [inp_CanValid_bus] -> slr1_16/1
  slr1_16/1 -> TFootRr/3  "<VINP_CANMsgValidZoneDrTHCM_flg>"
  TFootRr/1 -> VINP_TFootRr_C/1  "VINP_TFootRr_C"
  TFootRr/2 -> Terminator_16/1
  [BHAL_outputs] -> slr_VHAL_TFootRrErr_enum/1
  slr_VHAL_TFootRrErr_enum/1 -> TFootRrErr/1  "<VHAL_TFootRrErr_enum>"
  True_VHAL_TFootRrErr_enum/1 -> TFootRrErr/2
  [inp_CanValid_bus] -> slr1_17/1
  slr1_17/1 -> TFootRrErr/3  "<VINP_CANMsgValidZoneDrTHCM_flg>"
  TFootRrErr/1 -> VINP_TFootRrErr_enum/1  "VINP_TFootRrErr_enum"
  TFootRrErr/2 -> Terminator_17/1
  [BHAL_outputs] -> slr_VHAL_Tevap_C/1
  slr_VHAL_Tevap_C/1 -> Tevap/1  "<VHAL_Tevap_C>"
  True_VHAL_Tevap_C/1 -> Tevap/2
  [inp_CanValid_bus] -> slr1_18/1
  slr1_18/1 -> Tevap/3  "<VINP_CANMsgValidZoneDrTHCM_flg>"
  Tevap/1 -> VINP_Tevap_C/1  "VINP_Tevap_C"
  Tevap/2 -> Terminator_18/1
  [BHAL_outputs] -> slr_VHAL_TevapErr_enum/1
  slr_VHAL_TevapErr_enum/1 -> TevapErr/1  "<VHAL_TevapErr_enum>"
  True_VHAL_TevapErr_enum/1 -> TevapErr/2
  [inp_CanValid_bus] -> slr1_19/1
  slr1_19/1 -> TevapErr/3  "<VINP_CANMsgValidZoneDrTHCM_flg>"
  TevapErr/1 -> VINP_TevapErr_enum/1  "VINP_TevapErr_enum"
  TevapErr/2 -> Terminator_19/1
  [BHAL_outputs] -> slr_VHAL_Tincar_C/1
  slr_VHAL_Tincar_C/1 -> Tincar/1  "<VHAL_Tincar_C>"
  True_VHAL_Tincar_C/1 -> Tincar/2
  [inp_CanValid_bus] -> slr1_20/1
  slr1_20/1 -> Tincar/3  "<VINP_CANMsgValidZoneDrTHCM_flg>"
  Tincar/1 -> VINP_Tincar_C/1  "VINP_Tincar_C"
  Tincar/2 -> Terminator_20/1
  [BHAL_outputs] -> slr_VHAL_TincarErr_enum/1
  slr_VHAL_TincarErr_enum/1 -> TincarErr/1  "<VHAL_TincarErr_enum>"
  True_VHAL_TincarErr_enum/1 -> TincarErr/2
  [inp_CanValid_bus] -> slr1_21/1
  slr1_21/1 -> TincarErr/3  "<VINP_CANMsgValidZoneDrTHCM_flg>"
  TincarErr/1 -> VINP_TincarErr_enum/1  "VINP_TincarErr_enum"
  TincarErr/2 -> Terminator_21/1
